simulink library "galipeur_lib"  (R2017a)
settings: Solver=VariableStepAuto  StartTime=0.0  StopTime=10.0  RelTol=1e-3
undefined symbols (not defined in the file): FXA315_radius, PLG32_factor, RE25_Ke, RE25_Kt, RE25_r
libraries: ccmotor_lib x1
settings Model: Creator=jdam  LastModifiedBy=jdam

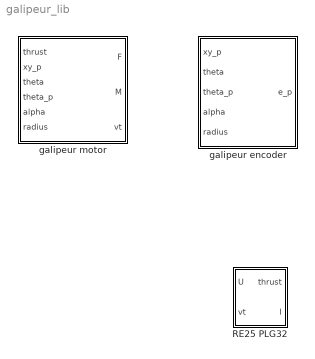
== system galipeur_lib ==
  RE25 PLG32 : Subsystem
  galipeur encoder : Subsystem
  galipeur motor : Subsystem

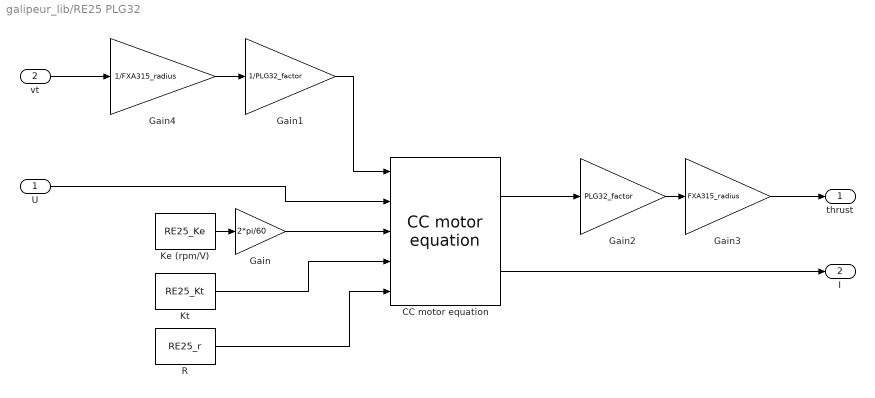
== system galipeur_lib/RE25 PLG32 ==
  U : Inport
  vt : Inport  Port=2
  CC motor equation : ccmotor_lib/CC motor equation
  Gain : Gain  Gain=2*pi/60
  Gain1 : Gain  Gain=1/PLG32_factor
  Gain2 : Gain  Gain=PLG32_factor
  Gain3 : Gain  Gain=FXA315_radius
  Gain4 : Gain  Gain=1/FXA315_radius
  Ke (rpm/V) : Constant  Value=RE25_Ke
  Kt : Constant  Value=RE25_Kt
  R : Constant  Value=RE25_r
  thrust : Outport
  I : Outport  Port=2
  wires:
  CC motor equation/1 -> Gain2/1
  Ke (rpm/V)/1 -> Gain/1
  Gain2/1 -> Gain3/1
  R/1 -> CC motor equation/5
  Kt/1 -> CC motor equation/4
  Gain3/1 -> thrust/1
  U/1 -> CC motor equation/2
  Gain1/1 -> CC motor equation/1
  Gain/1 -> CC motor equation/3
  CC motor equation/2 -> I/1
  Gain4/1 -> Gain1/1
  vt/1 -> Gain4/1

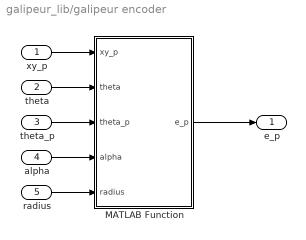
== system galipeur_lib/galipeur encoder ==
  xy_p : Inport
  theta : Inport  Port=2
  theta_p : Inport  Port=3
  alpha : Inport  Port=4
  radius : Inport  Port=5
  MATLAB Function : MATLAB Function  TreatAsAtomicUnit=on
  e_p : Outport
  wires:
  xy_p/1 -> MATLAB Function/1(xy_p)
  theta/1 -> MATLAB Function/2(theta)
  theta_p/1 -> MATLAB Function/3(theta_p)
  alpha/1 -> MATLAB Function/4(alpha)
  radius/1 -> MATLAB Function/5(radius)
  MATLAB Function/1(e_p) -> e_p/1

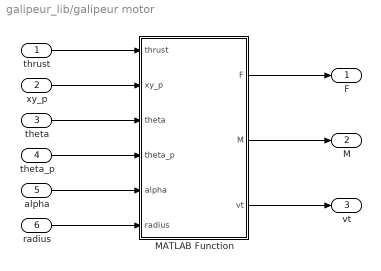
== system galipeur_lib/galipeur motor ==
  thrust : Inport
  xy_p : Inport  Port=2
  theta : Inport  Port=3
  theta_p : Inport  Port=4
  alpha : Inport  Port=5
  radius : Inport  Port=6
  MATLAB Function : MATLAB Function  TreatAsAtomicUnit=on
  F : Outport
  M : Outport  Port=2
  vt : Outport  Port=3
  wires:
  thrust/1 -> MATLAB Function/1(thrust)
  xy_p/1 -> MATLAB Function/2(xy_p)
  theta/1 -> MATLAB Function/3(theta)
  theta_p/1 -> MATLAB Function/4(theta_p)
  alpha/1 -> MATLAB Function/5(alpha)
  radius/1 -> MATLAB Function/6(radius)
  MATLAB Function/1(F) -> F/1
  MATLAB Function/2(M) -> M/1
  MATLAB Function/3(vt) -> vt/1

== matlab function galipeur_lib/galipeur encoder/MATLAB Function ==
  data: xy_p input; e_p output; theta input; theta_p input; alpha input; radius input
function e_p = fcn(xy_p,theta,theta_p,alpha,radius)
% xy_p: robot velocity in ground reference (xp, yp)
% alpha: motor orientation placement relative to robot
% radius: motor distance from robot CG relative to robot
% theta: robot orientation relative to ground
% theta_p: robot rotation speed

% compute unitary vector perpendicular to thrust
up = [cos(theta+alpha); sin(theta+alpha)];
% compute unitary vector along thrust
ut = [-sin(theta+alpha); cos(theta+alpha)];

% transport speed to contact point
vm = xy_p + radius*theta_p*ut;

% project speed onto unitary thrust vector
e_p = dot(vm,ut);

== matlab function galipeur_lib/galipeur motor/MATLAB Function ==
  data: thrust input; F output; xy_p input; theta input; theta_p input; alpha input; radius input; M output; vt output
function [F,M,vt]= fcn(thrust, xy_p, theta, theta_p, alpha, radius)
% thrust: motor thrust in N at contact
% xy_p: robot velocity in ground reference (xp, yp)
% alpha: motor orientation placement relative to robot
% radius: motor distance from robot CG relative to robot
% theta: robot orientation relative to ground
% theta_p: robot rotation speed

% compute unitary vector perpendicular to thrust
up = [cos(theta+alpha); sin(theta+alpha)];
% compute unitary vector along thrust
ut = [-sin(theta+alpha); cos(theta+alpha)];

% transport velocity to contact point
vm = xy_p + radius*theta_p*ut;

% project velocity along thrust (in motor)
vt = dot(vm,ut);
% project velocity perpendicular to thrust (rolling omniwheel)
vp = dot(vm,up);

% omniwheel rolling friction
fp = 0.01;

% compute sum of forces for this motor
F = thrust*ut - vp*fp;
% compute momentum at robot CoG 
GM = up*radius;
momentum = cross([GM(1);GM(2);0],[F(1);F(2);0]);
M = momentum(3);
